simulink model "model2_cm"  (R2018b)
settings: Solver=ode8  StartTime=0.0  StopTime=0  FixedStep=0.01  RelTol=1e-3  EnableMultiTasking=on
StopFcn:
  | % stopCallback
undefined symbols (not defined in the file): ipaddr, PTP
libraries: xpcutilitieslib x3, xpcrtudplib x3, ptplib x1
settings Model: sg_rtwmakecfg_data=_sglibc_  Creator=mcobb  LastModifiedBy=mcobb
settings SolverCC: ConcurrentTasks=on  AutoInsertRateTranBlk=on
settings DataIOCC: SaveFormat=StructureWithTime
settings OptimizationCC: BlockReduction=off  UseFloatMulNetSlope=on  EnhancedBackFolding=on  PassReuseOutputArgsThreshold=0  EfficientFloat2IntCast=on  OptimizeBlockOrder=speed  DifferentSizesBufferReuse=on  OptimizationCustomize=off
settings DebuggingCC: ParameterOverflowMsg=none  ParameterTunabilityLossMsg=error  LibraryContextMissingDiagnostic=none  UnitsInconsistencyMsg=none
settings HardwareCC: ProdBitPerPointer=32  ProdBitPerSizeT=32  ProdBitPerPtrDiffT=32  ProdLargestAtomicFloat=None  ProdWordSize=32  ProdLongLongMode=on  ProdHWDeviceType=Generic->32-bit x86 compatible
settings SFSimCC: SimUseLocalCustomCode=off  MATLABDynamicMemAlloc=off
settings RTWCC: SystemTargetFile=slrt.tlc  TLCOptions=-axPCMaxOverloads=2000  TemplateMakefile=slrt_default_tmf  Description=Simulink Real-Time  RTWUseLocalCustomCode=off  BuildConfiguration=Debug  CodeExecutionProfiling=on  RTWCompilerOptimization=on
settings CodeAppCC: ForceParamTrailComments=on  OperatorAnnotations=on
settings SimulinkRealTimeCC: SupportVariableSizeSignals=on  PreserveStateflowLocalDataDimensions=off  RL32ObjectName=tg2  xPCisDefaultEnv=off  xPCTargetPCEnvName=Machine2  xPCConcurrentTasks=on

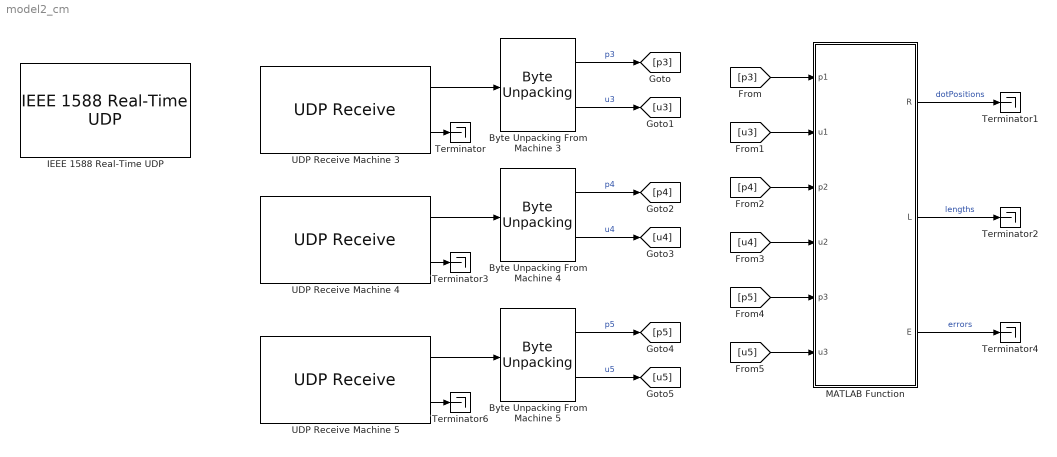
== system model2_cm ==
  "Byte Unpacking From Machine 3 " : xpcutilitieslib/Byte Unpacking   MaskUnpackedDataTypes={['double'],['double']}  MaskUnpackedDataSizes={[27],[27]}  MaskAlignment=1
      settings: SourceProductName=Simulink Real-Time  SourceProductBaseCode=XP
  Byte Unpacking From Machine 4 : xpcutilitieslib/Byte Unpacking   MaskUnpackedDataTypes={['double'],['double']}  MaskUnpackedDataSizes={[27],[27]}  MaskAlignment=1
      settings: SourceProductName=Simulink Real-Time  SourceProductBaseCode=XP
  Byte Unpacking From Machine 5 : xpcutilitieslib/Byte Unpacking   MaskUnpackedDataTypes={['double'],['double']}  MaskUnpackedDataSizes={[27],[27]}  MaskAlignment=1
      settings: SourceProductName=Simulink Real-Time  SourceProductBaseCode=XP
  IEEE 1588 Real-Time UDP : ptplib/IEEE 1588 Real-Time UDP  Priority=0  ID=1  PciBus=2  PciSlot=0  PciFunction=0  time_inc=4000000  sample_time=-1  IpSource=Specify  IpAddress=30.30.30.30  SubnetMask=255.255.255.0  Gateway=0.0.0.0  Receive1=0.0.0.0  dest_ip_select=Specify  custom_dest_ip_addr=255.255.255.255  MulticastList=[ipaddr('224.0.1.129'), ipaddr('224.0.0.107')]  Multicast={macaddr('01:00:5E:00:01:81'), macaddr('01:00:5E:00:00:6B')}  time_source=Ethernet board  timescale=PTP (1970-01-01)  epoch=[1970 01 01 00]  delay_measure=Request-response  slave_only=off  enable_advanced_config=on  domain_num=0  utc_offset=35  priority1=1  clock_class=248  clock_accuracy=hex2dec('FE')  priority2=1  announce_interval=1  sync_interval=0.1  min_pdelay_req_interval=2  announce_receipt_timeout=5
      settings: SourceProductName=Simulink Real-Time  SourceProductBaseCode=XP
  MATLAB Function : MATLAB Function  TreatAsAtomicUnit=on
  Terminator{,1..4,6} (6 alike) : Terminator
  UDP Receive Machine 3 : xpcrtudplib/UDP Receive  ipAddressVal=30.30.30.30  localPort=8002  rcvWidth=32  rcvFmAny=off  fmAddress=30.30.30.1  rcvMulticast=off  multicastAddress={30.30.30.1, 30.30.30.2, 30.30.30.3}  maxUDPQueue=8  sampleTime=-1
      settings: SourceProductName=Simulink Real-Time
  UDP Receive Machine 4 : xpcrtudplib/UDP Receive  ipAddressVal=Use host-target connection  localPort=8002  rcvWidth=32  rcvFmAny=off  fmAddress=30.30.30.2  rcvMulticast=off  multicastAddress={30.30.30.1, 30.30.30.2, 30.30.30.3}  maxUDPQueue=8  sampleTime=sample_time
      settings: SourceProductName=Simulink Real-Time
  UDP Receive Machine 5 : xpcrtudplib/UDP Receive  ipAddressVal=30.30.30.30  localPort=8002  rcvWidth=32  rcvFmAny=off  fmAddress=30.30.30.3  rcvMulticast=off  multicastAddress={30.30.30.1, 30.30.30.2, 30.30.30.3}  maxUDPQueue=8  sampleTime=-1
      settings: SourceProductName=Simulink Real-Time
  wires:
  UDP Receive Machine 3/1 -> "Byte Unpacking From Machine 3 "/1
  UDP Receive Machine 3/2 -> Terminator/1
  Byte Unpacking From Machine 4/2 -> [u4]  "u4"
  Byte Unpacking From Machine 4/1 -> [p4]  "p4"
  UDP Receive Machine 4/2 -> Terminator3/1
  UDP Receive Machine 4/1 -> Byte Unpacking From Machine 4/1
  UDP Receive Machine 5/1 -> Byte Unpacking From Machine 5/1
  UDP Receive Machine 5/2 -> Terminator6/1
  Byte Unpacking From Machine 5/1 -> [p5]  "p5"
  Byte Unpacking From Machine 5/2 -> [u5]  "u5"
  "Byte Unpacking From Machine 3 "/1 -> [p3]  "p3"
  "Byte Unpacking From Machine 3 "/2 -> [u3]  "u3"
  [p3] -> MATLAB Function/1(p1)
  [u3] -> MATLAB Function/2(u1)
  [p4] -> MATLAB Function/3(p2)
  [u4] -> MATLAB Function/4(u2)
  [p5] -> MATLAB Function/5(p3)
  [u5] -> MATLAB Function/6(u3)
  MATLAB Function/1(R) -> Terminator1/1  "dotPositions"
  MATLAB Function/2(L) -> Terminator2/1  "lengths"
  MATLAB Function/3(E) -> Terminator4/1  "errors"

== matlab function model2_cm/MATLAB Function ==
  data: R output; p1 input; u1 input; p2 input; u2 input; p3 input; u3 input; L output; E output
function [R,L,E] = fcn(p1,u1,p2,u2,p3,u3)
% Function to calculate the least squares solution for the position of the
% dots being tracked on machines 3, 4, and 5.
% In this documentation:
% N is the number of dots being tracked.
% i is an index that runs from 1 to N and refers to which dot is being
% tracked.
% j is an index that runs from 1 to 3 and refers to which camera is being
% considered.  Note that camera 1 is attached to machine 3, camera 2 is
% attached to machine 4, and camera 3 is attached to machine 5.
% O is the point at the origin of the "inertial" or ground-fixed coordinate
% system.

% INPUTS
% pj is a 3 by N matrix of points produced by the ray tracing algorithm
% associated with camera j.
% uj is a 3 by N matrix of unit vectors produced by the ray tracing
% algorithm associated with camera j.

% OUTPUTS
% R is a 3 by N matrix of the estimated position vectors of each dot.
% L is a 3 by N row vector of the scalar lengths along each unit vector
% that best fit the observed data.
% E is a 1 by N vector of squared error terms (E(3) is the sum of squared
% squared errors for the position of dot 3).

% A sketchy whiteboard derivation of this method is provided in
% ./Documentation/LeastSquaresSolution.jpg

% Preallocate the outputs, simulink needs this to figure out the dimensions
% of the output signals.
L = zeros(3,size(p1,2));
R = ones(3,size(p1,2));
E = zeros(1,size(p1,2));

% Calculate the A matrix.
A = [...
    eye(3)      -eye(3)     zeros(3,3)  ;...
    eye(3)      zeros(3,3)  -eye(3)     ;...
    zeros(3,3)  eye(3,3)    -eye(3,3)   ];
% Calculate intermediate variable so the loop doesn't have to do this
% repeatedly
A0 = A'*A;

% Concatenate input position vector matrices vertically
P0 = [p1;p2;p3];

% Loop over every combination of points and unit vectors
for ii = 1:size(p1,2)
    % Build the matrix U_i
    Ui = [...
        u1(:,ii)     zeros(3,1)  zeros(3,1);...
        zeros(3,1)   u2(:,ii)    zeros(3,1);...
        zeros(3,1)   zeros(3,1)  u3(:,ii)];
    % Calculate the lengths along the unit vectors via least squares
    Li = -inv(Ui'*A0*Ui)*Ui'*A0*P0(:,ii);
    % Save the results into the output matrix
    L(:,ii) = Li(:);
    % Calculate the resulting dot positions
    Ri = P0(:,ii) + Ui*Li(:);
    % Average the three results
    R(:,ii) = (Ri(1:3) + Ri(4:6) + Ri(7:9))/3;
    % Calculate sum of squared errors for this dot
    E(ii) = Ri(:)'*A0*Ri(:);
end

end
